simulink model "DengFOC"  (R2022a)
settings: Solver=VariableStepAuto  StartTime=0.0  StopTime=1  RelTol=1e-3
libraries: simulink x1
settings Model: Creator=Mengyang  LastModifiedBy=Mengyang

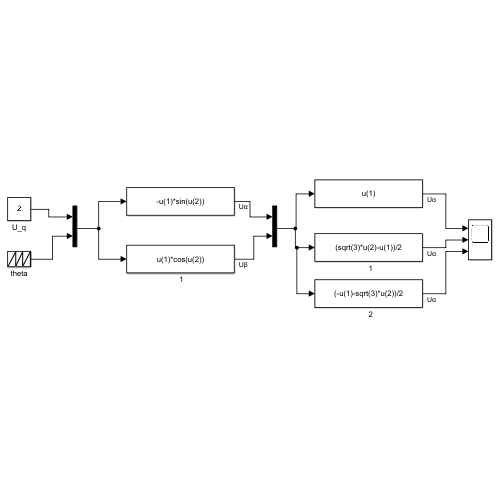
[thumbnail: Simulink's stored preview of the top-level diagram]
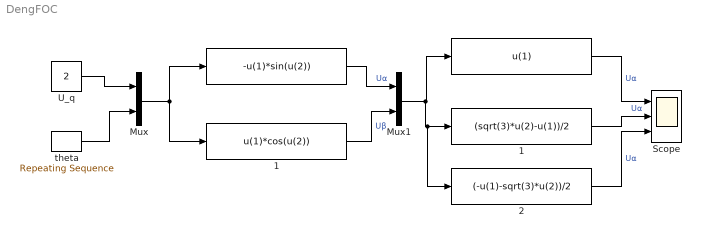
== system DengFOC ==
  " " : Fcn  Expr=-u(1)*sin(u(2))
  "  " : Fcn  Expr=u(1)
  "  1" : Fcn  Expr=(sqrt(3)*u(2)-u(1))/2
  "  2" : Fcn  Expr=(-u(1)-sqrt(3)*u(2))/2
  " 1" : Fcn  Expr=u(1)*cos(u(2))
  Mux : Mux  Inputs=2
  Mux1 : Mux  Inputs=2
  Scope : Scope  NumInputPorts=3
  U_q : Constant  Value=2
  "theta " : simulink/Sources/Repeating Sequence  rep_seq_t=[0 1]  rep_seq_y=[0 2*pi]
  wires:
  U_q/1 -> Mux/1
  "theta "/1 -> Mux/2
  Mux/1 -> " 1"/1, " "/1
  " "/1 -> Mux1/1  "Uα"
  " 1"/1 -> Mux1/2  "Uβ"
  Mux1/1 -> "  2"/1, "  1"/1, "  "/1
  "  "/1 -> Scope/1  "Uα"
  "  1"/1 -> Scope/2  "Uα"
  "  2"/1 -> Scope/3  "Uα"
